simulink model "PotenSchmittwSTM"  (R2024b)
settings: Solver=FixedStepAuto  StartTime=0.0  StopTime=inf  RelTol=1e-3  EnableMultiTasking=on
libraries: fl_lib x16, nesl_utility x10, stm32f4xxblockslib x1
settings Model: STM32="{\"AnalogInput\":[{\"ID\":\"Poten1:1\"},{\"ID\":\"PotenSchmittwSTM:1\"}]}"  Creator=pongn  LastModifiedBy=pongn
settings OptimizationCC: DefaultParameterBehavior=Inlined  EnhancedBackFolding=on  PassReuseOutputArgsAs=Individual arguments  ZeroExternalMemoryAtStartup=off  ZeroInternalMemoryAtStartup=off  MaxStackSize=512  OptimizeBlockOrder=speed  DifferentSizesBufferReuse=on  OptimizationCustomize=off  EfficientTunableParamExpr=on
settings DebuggingCC: ParameterTunabilityLossMsg=error
settings HardwareCC: ProdBitPerPointer=32  ProdBitPerSizeT=32  ProdBitPerPtrDiffT=32  ProdLargestAtomicInteger=Long  ProdLargestAtomicFloat=Double  ProdWordSize=32  ProdLongLongMode=on  ProdHWDeviceType=ARM Compatible->ARM Cortex-M
settings SFSimCC: MATLABDynamicMemAlloc=off
settings RTWCC: Description=Embedded Coder  SystemTargetFile=ert.tlc  HardwareBoard=STM32G4xx Based  TemplateMakefile=ert_default_tmf  Toolchain=GNU Tools for ARM Embedded Processors
settings CodeAppCC: ForceParamTrailComments=on  IgnoreCustomStorageClasses=off  OperatorAnnotations=on  SimulinkDataObjDesc=on  SFDataObjDesc=on  InsertBlockDesc=on
settings ERTTargetCC: TargetLangStandard=C99 (ISO)  CodeReplacementLibrary=ARM Cortex-M  ExtModeTransport=3  ExtModeStaticAlloc=on  ExtModeStaticAllocSize=2048  ExtModeMexFile=ext_xcp  ExtModeIntrfLevel=Level2 - Open

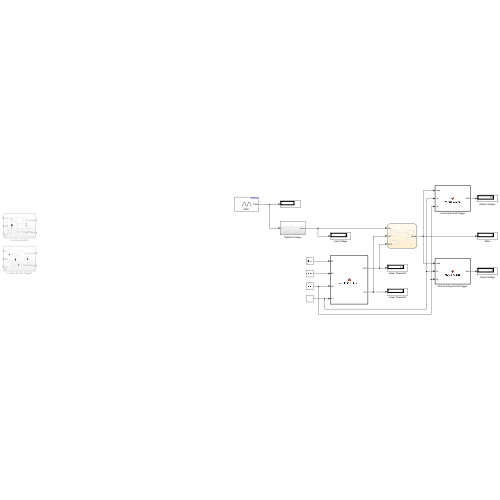
[thumbnail: Simulink's stored preview of the top-level diagram]
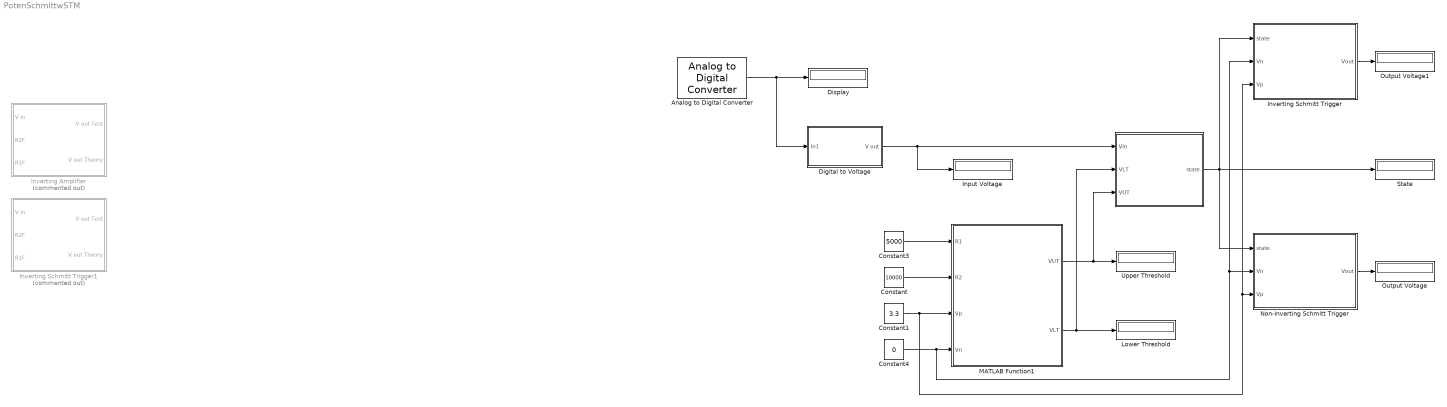
== system PotenSchmittwSTM ==
  " " : Stateflow chart  TreatAsAtomicUnit=on
  Analog to Digital Converter : stm32f4xxblockslib/Analog to Digital Converter  ADCModule=ADC1  ConversionGroup=Regular  TriggerMode=Trigger and read  NumberOfConversions=1  EnableBufferConv=off  BufferLength=1  OutputStatus=off  SampleTime=-1  EnableSimPort=off  hoistedMaskSrc=ECSoC/ECSimCodegen/Analog to Digital Converter
  Constant : Constant  Value=10000
  Constant1 : Constant  Value=3.3
  Constant3 : Constant  Value=5000
  Constant4 : Constant  Value=0
  Digital to Voltage : Subsystem
  Display : Display
  Input Voltage : Display
  Inverting Amplifier : Subsystem  Commented=on
  Inverting Schmitt Trigger : MATLAB Function  TreatAsAtomicUnit=on
  Inverting Schmitt Trigger1 : Subsystem  Commented=on
  Lower Threshold : Display
  MATLAB Function1 : MATLAB Function  TreatAsAtomicUnit=on
  Non-Inverting Schmitt Trigger : MATLAB Function  TreatAsAtomicUnit=on
  Output Voltage : Display
  Output Voltage1 : Display
  State : Display
  Upper Threshold : Display
  wires:
  Analog to Digital Converter/1 -> Digital to Voltage/1(In1), Display/1
  " "/1(state) -> Inverting Schmitt Trigger/1(state), State/1, Non-Inverting Schmitt Trigger/1(state)
  Constant3/1 -> MATLAB Function1/1(R1)
  Constant/1 -> MATLAB Function1/2(R2)
  Constant4/1 -> MATLAB Function1/4(Vn), Inverting Schmitt Trigger/2(Vn), Non-Inverting Schmitt Trigger/2(Vn)
  MATLAB Function1/1(VUT) -> " "/3(VUT), Upper Threshold/1
  MATLAB Function1/2(VLT) -> " "/2(VLT), Lower Threshold/1
  Constant1/1 -> Inverting Schmitt Trigger/3(Vp), Non-Inverting Schmitt Trigger/3(Vp), MATLAB Function1/3(Vp)
  Non-Inverting Schmitt Trigger/1(Vout) -> Output Voltage/1
  Inverting Schmitt Trigger/1(Vout) -> Output Voltage1/1
  Digital to Voltage/1(V out) -> Input Voltage/1, " "/1(Vin)

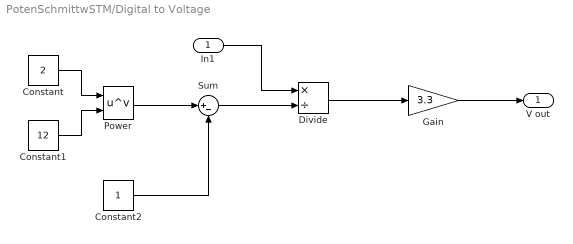
== system PotenSchmittwSTM/Digital to Voltage ==
  In1 : Inport
  Constant : Constant  Value=2
  Constant1 : Constant  Value=12
  Constant2 : Constant
  Divide : Product  Inputs=*/
  Gain : Gain  Gain=3.3
  Power : Math  Operator=pow
  Sum : Sum  Inputs=|+-
  V out : Outport
  wires:
  Constant/1 -> Power/1
  Constant2/1 -> Sum/2
  Sum/1 -> Divide/2
  Power/1 -> Sum/1
  Divide/1 -> Gain/1
  Constant1/1 -> Power/2
  Gain/1 -> V out/1
  In1/1 -> Divide/1

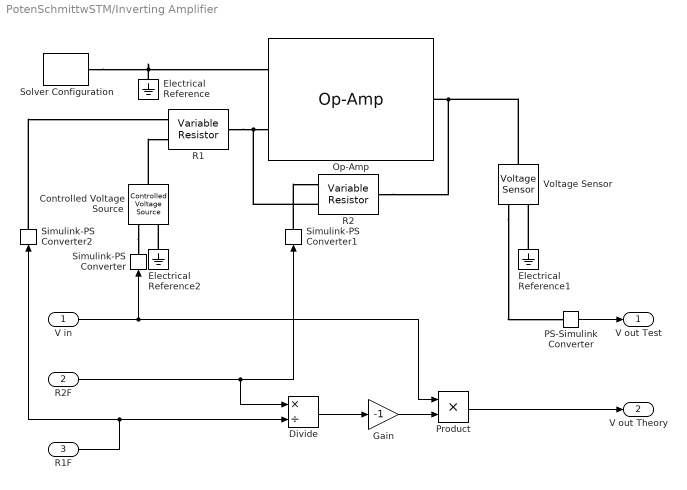
== system PotenSchmittwSTM/Inverting Amplifier ==
  V in : Inport
  R2F : Inport  Port=2
  R1F : Inport  Port=3
  Controlled Voltage Source : fl_lib/Electrical/Electrical Sources/Controlled Voltage Source
  Divide : Product  Inputs=*/
  Electrical Reference : fl_lib/Electrical/Electrical Elements/Electrical Reference
  Electrical Reference1 : fl_lib/Electrical/Electrical Elements/Electrical Reference
  Electrical Reference2 : fl_lib/Electrical/Electrical Elements/Electrical Reference
  Gain : Gain  Gain=-1
  Op-Amp : fl_lib/Electrical/Electrical Elements/Op-Amp  outI_specify=off  outI_priority=None  outI=0 A  outI_nominal_specify=off  outI_nominal_value=1  outI_nominal_unit=A
  PS-Simulink Converter : nesl_utility/PS-Simulink Converter  PhysicalDomain=network_engine_domain  SubClassName=ps_output  LeftPortType=input  RightPortType=output  PseudoPeriodic=off  Frequencies=[]  VectorFormat=inherit  Unit=inherit  AffineConversion=off
  Product : Product
  R1 : fl_lib/Electrical/Electrical Elements/Variable Resistor  Rmin=0 Ohm  thermalEnable=false  thermal_mass=1 J/K  i_specify=off  i_priority=None  i=0 A  i_nominal_specify=off  i_nominal_value=1  i_nominal_unit=A  v_specify=off  v_priority=None  v=0 V  v_nominal_specify=off  v_nominal_value=1  v_nominal_unit=V  T_specify=off  T_priority=None  T=300 K  T_nominal_specify=off  T_nominal_value=1  T_nominal_unit=K
  R2 : fl_lib/Electrical/Electrical Elements/Variable Resistor  Rmin=0 Ohm  thermalEnable=false  thermal_mass=1 J/K  i_specify=off  i_priority=None  i=0 A  i_nominal_specify=off  i_nominal_value=1  i_nominal_unit=A  v_specify=off  v_priority=None  v=0 V  v_nominal_specify=off  v_nominal_value=1  v_nominal_unit=V  T_specify=off  T_priority=None  T=300 K  T_nominal_specify=off  T_nominal_value=1  T_nominal_unit=K
  Simulink-PS Converter : nesl_utility/Simulink-PS Converter  PhysicalDomain=network_engine_domain  SubClassName=ps_input  LeftPortType=input  RightPortType=output  PseudoPeriodic=off  Frequencies=[]  NoiseDistribution=none  NoiseParameters=[]  Unit=1  AffineConversion=off  FilteringAndDerivatives=provide  SimscapeFilterOrder=1  InputFilterTimeConstant=0.001  UdotUserProvided=0
  Simulink-PS Converter1 : nesl_utility/Simulink-PS Converter  PhysicalDomain=network_engine_domain  SubClassName=ps_input  LeftPortType=input  RightPortType=output  PseudoPeriodic=off  Frequencies=[]  NoiseDistribution=none  NoiseParameters=[]  Unit=1  AffineConversion=off  FilteringAndDerivatives=provide  SimscapeFilterOrder=1  InputFilterTimeConstant=0.001  UdotUserProvided=0
  Simulink-PS Converter2 : nesl_utility/Simulink-PS Converter  PhysicalDomain=network_engine_domain  SubClassName=ps_input  LeftPortType=input  RightPortType=output  PseudoPeriodic=off  Frequencies=[]  NoiseDistribution=none  NoiseParameters=[]  Unit=1  AffineConversion=off  FilteringAndDerivatives=provide  SimscapeFilterOrder=1  InputFilterTimeConstant=0.001  UdotUserProvided=0
  Solver Configuration : nesl_utility/Solver Configuration  PhysicalDomain=network_engine_domain  SubClassName=solver  LeftPortType=input  RightPortType=generic  Tones=[]  Harmonics=[]  SimulateNoise=off  Profile=off  UseLocalSampling=off  EnableSwitchedLinearOptims=on  FrequencyDomain=off  UseCCode=off  RelTol=0.001  AbsTol=0.001  MinStep=1e-09  ToWorkspace=off  RevertToSquareIcSolve=off  NumHomotopyIterations=100  PhasorMode=off  PhasorModeNumHarmonics=1  ConsistencySolver=NEWTON_XTOL_AFTER_FTOL  IndexReductionMethod=DerivativeReplacement  DoDC=off  ResidualTolerance=1e-09  ConsistencyTolSource=GLOBAL  ConsistencyAbsTol=0.001  ConsistencyRelTol=0.001  ConsistencyTolFactor=0.001  UseLocalSolver=off  LocalSolverChoice=NE_BACKWARD_EULER_ADVANCER  ResolveIndetEquations=on  FunctionEvalNumThread=1  LocalSolverSampleTime=0.001  DoFixedCost=off  MaxNonlinIter=3  MaxModeIter=2  ComputeImpulses=off  ImpulseIterations=2  LinearAlgebra=auto  LinearAlgebraNumThread=0  EquationFormulation=NE_TIME_EF  DelaysMemoryBudget=1024  AutomaticFiltering=on  FilteringTimeConstant=0.001  PartitionStorageMethod=AS_NEEDED  PartitionMemoryBudget=1024  PartitionMethod=ROBUST  MultibodyUseLocalSolver=off  MultibodyLocalSolverChoice=ODE1  MultibodyLocalSolverSampleTime=0.001
  Voltage Sensor : fl_lib/Electrical/Electrical Sensors/Voltage Sensor
  V out Test : Outport
  V out Theory : Outport  Port=2
  wires:
  Divide/1 -> Gain/1
  Gain/1 -> Product/2
  V in/1 -> Simulink-PS Converter/1, Product/1
  Product/1 -> V out Theory/1
  R2F/1 -> Simulink-PS Converter1/1, Divide/1
  R1F/1 -> Divide/2, Simulink-PS Converter2/1
  PS-Simulink Converter/1 -> V out Test/1
  connections:
  Voltage Sensor/LConn1 -- Op-Amp/RConn1 -- R2/RConn1
  R1/RConn1 -- Op-Amp/LConn2 -- R2/LConn2
  Solver Configuration/RConn1 -- Electrical Reference/LConn1 -- Op-Amp/LConn1
  Voltage Sensor/RConn1 -- PS-Simulink Converter/LConn1
  Electrical Reference1/LConn1 -- Voltage Sensor/RConn2
  Controlled Voltage Source/RConn1 -- Simulink-PS Converter/RConn1
  Controlled Voltage Source/LConn1 -- R1/LConn2
  Electrical Reference2/LConn1 -- Controlled Voltage Source/RConn2
  Simulink-PS Converter1/RConn1 -- R2/LConn1
  Simulink-PS Converter2/RConn1 -- R1/LConn1

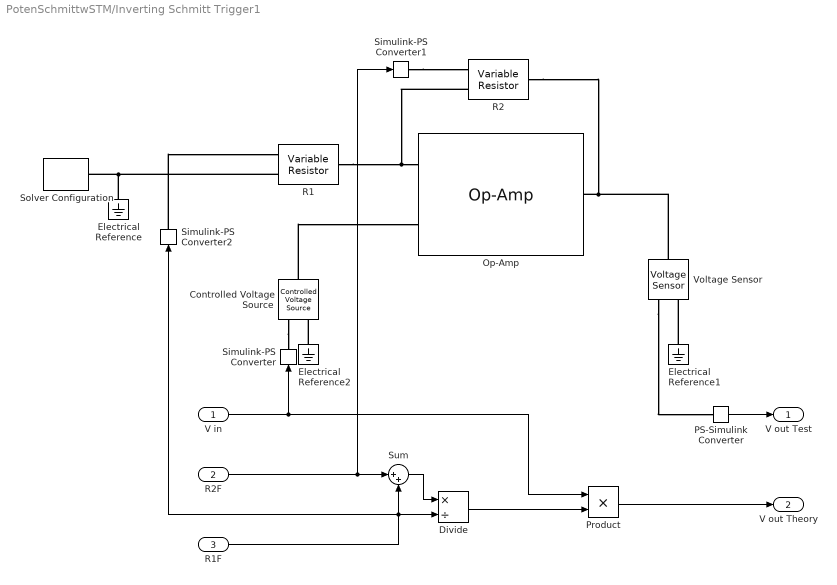
== system PotenSchmittwSTM/Inverting Schmitt Trigger1 ==
  V in : Inport
  R2F : Inport  Port=2
  R1F : Inport  Port=3
  Controlled Voltage Source : fl_lib/Electrical/Electrical Sources/Controlled Voltage Source
  Divide : Product  Inputs=*/
  Electrical Reference : fl_lib/Electrical/Electrical Elements/Electrical Reference
  Electrical Reference1 : fl_lib/Electrical/Electrical Elements/Electrical Reference
  Electrical Reference2 : fl_lib/Electrical/Electrical Elements/Electrical Reference
  Op-Amp : fl_lib/Electrical/Electrical Elements/Op-Amp  outI_specify=off  outI_priority=None  outI=0 A  outI_nominal_specify=off  outI_nominal_value=1  outI_nominal_unit=A
  PS-Simulink Converter : nesl_utility/PS-Simulink Converter  PhysicalDomain=network_engine_domain  SubClassName=ps_output  LeftPortType=input  RightPortType=output  PseudoPeriodic=off  Frequencies=[]  VectorFormat=inherit  Unit=inherit  AffineConversion=off
  Product : Product
  R1 : fl_lib/Electrical/Electrical Elements/Variable Resistor  Rmin=0 Ohm  thermalEnable=false  thermal_mass=1 J/K  i_specify=off  i_priority=None  i=0 A  i_nominal_specify=off  i_nominal_value=1  i_nominal_unit=A  v_specify=off  v_priority=None  v=0 V  v_nominal_specify=off  v_nominal_value=1  v_nominal_unit=V  T_specify=off  T_priority=None  T=300 K  T_nominal_specify=off  T_nominal_value=1  T_nominal_unit=K
  R2 : fl_lib/Electrical/Electrical Elements/Variable Resistor  Rmin=0 Ohm  thermalEnable=false  thermal_mass=1 J/K  i_specify=off  i_priority=None  i=0 A  i_nominal_specify=off  i_nominal_value=1  i_nominal_unit=A  v_specify=off  v_priority=None  v=0 V  v_nominal_specify=off  v_nominal_value=1  v_nominal_unit=V  T_specify=off  T_priority=None  T=300 K  T_nominal_specify=off  T_nominal_value=1  T_nominal_unit=K
  Simulink-PS Converter : nesl_utility/Simulink-PS Converter  PhysicalDomain=network_engine_domain  SubClassName=ps_input  LeftPortType=input  RightPortType=output  PseudoPeriodic=off  Frequencies=[]  NoiseDistribution=none  NoiseParameters=[]  Unit=1  AffineConversion=off  FilteringAndDerivatives=provide  SimscapeFilterOrder=1  InputFilterTimeConstant=0.001  UdotUserProvided=0
  Simulink-PS Converter1 : nesl_utility/Simulink-PS Converter  PhysicalDomain=network_engine_domain  SubClassName=ps_input  LeftPortType=input  RightPortType=output  PseudoPeriodic=off  Frequencies=[]  NoiseDistribution=none  NoiseParameters=[]  Unit=1  AffineConversion=off  FilteringAndDerivatives=provide  SimscapeFilterOrder=1  InputFilterTimeConstant=0.001  UdotUserProvided=0
  Simulink-PS Converter2 : nesl_utility/Simulink-PS Converter  PhysicalDomain=network_engine_domain  SubClassName=ps_input  LeftPortType=input  RightPortType=output  PseudoPeriodic=off  Frequencies=[]  NoiseDistribution=none  NoiseParameters=[]  Unit=1  AffineConversion=off  FilteringAndDerivatives=provide  SimscapeFilterOrder=1  InputFilterTimeConstant=0.001  UdotUserProvided=0
  Solver Configuration : nesl_utility/Solver Configuration  PhysicalDomain=network_engine_domain  SubClassName=solver  LeftPortType=input  RightPortType=generic  Tones=[]  Harmonics=[]  SimulateNoise=off  Profile=off  UseLocalSampling=off  EnableSwitchedLinearOptims=on  FrequencyDomain=off  UseCCode=off  RelTol=0.001  AbsTol=0.001  MinStep=1e-09  ToWorkspace=off  RevertToSquareIcSolve=off  NumHomotopyIterations=100  PhasorMode=off  PhasorModeNumHarmonics=1  ConsistencySolver=NEWTON_XTOL_AFTER_FTOL  IndexReductionMethod=DerivativeReplacement  DoDC=off  ResidualTolerance=1e-09  ConsistencyTolSource=GLOBAL  ConsistencyAbsTol=0.001  ConsistencyRelTol=0.001  ConsistencyTolFactor=0.001  UseLocalSolver=off  LocalSolverChoice=NE_BACKWARD_EULER_ADVANCER  ResolveIndetEquations=on  FunctionEvalNumThread=1  LocalSolverSampleTime=0.001  DoFixedCost=off  MaxNonlinIter=3  MaxModeIter=2  ComputeImpulses=off  ImpulseIterations=2  LinearAlgebra=auto  LinearAlgebraNumThread=0  EquationFormulation=NE_TIME_EF  DelaysMemoryBudget=1024  AutomaticFiltering=on  FilteringTimeConstant=0.001  PartitionStorageMethod=AS_NEEDED  PartitionMemoryBudget=1024  PartitionMethod=ROBUST  MultibodyUseLocalSolver=off  MultibodyLocalSolverChoice=ODE1  MultibodyLocalSolverSampleTime=0.001
  Sum : Sum  Inputs=|++
  Voltage Sensor : fl_lib/Electrical/Electrical Sensors/Voltage Sensor
  V out Test : Outport
  V out Theory : Outport  Port=2
  wires:
  R2F/1 -> Simulink-PS Converter1/1, Sum/1
  Sum/1 -> Divide/1
  R1F/1 -> Divide/2, Simulink-PS Converter2/1, Sum/2
  PS-Simulink Converter/1 -> V out Test/1
  Product/1 -> V out Theory/1
  V in/1 -> Product/1, Simulink-PS Converter/1
  Divide/1 -> Product/2
  connections:
  Controlled Voltage Source/LConn1 -- Op-Amp/LConn2
  R2/LConn2 -- R1/RConn1 -- Op-Amp/LConn1
  Simulink-PS Converter2/RConn1 -- R1/LConn1
  Simulink-PS Converter1/RConn1 -- R2/LConn1
  Electrical Reference2/LConn1 -- Controlled Voltage Source/RConn2
  Controlled Voltage Source/RConn1 -- Simulink-PS Converter/RConn1
  Electrical Reference1/LConn1 -- Voltage Sensor/RConn2
  Voltage Sensor/RConn1 -- PS-Simulink Converter/LConn1
  R1/LConn2 -- Solver Configuration/RConn1 -- Electrical Reference/LConn1
  R2/RConn1 -- Op-Amp/RConn1 -- Voltage Sensor/LConn1

== matlab function PotenSchmittwSTM/MATLAB Function1 ==
  data: R1 input; R2 input; Vp input; VUT output; Vn input; VLT output
% VUT : Upper Threshold Voltage
% VLT : Lower Threshold Voltage
% Vout : Output Voltage
% Vin : Input Voltage
% R1 : 1st Resistor
% R2 : 2nd Resistor
% Vp : Op-Amp V+
% Vn : Op-Amp V-

function [VUT, VLT] = VariableCalculation(R1,R2,Vp, Vn)

VUT = Vp * (R2 / (R1 + R2));
VLT = Vn * (R2 / (R1 + R2));

== matlab function PotenSchmittwSTM/Non-Inverting Schmitt Trigger ==
  data: state input; Vn input; Vp input; Vout output
% VUT : Upper Threshold Voltage
% VLT : Lower Threshold Voltage
% Vout : Output Voltage
% Vin : Input Voltage
% R1 : 1st Resistor
% R2 : 2nd Resistor
% Vp : Op-Amp V+
% Vn : Op-Amp V-

function Vout = VoutCalculation(state, Vn, Vp)
Vout = 0;

if state == 1
    Vout = Vp;
elseif state == 0
    Vout = Vn;
end

== stateflow chart PotenSchmittwSTM/  ==
  state Initial
    state = 0;
  state LessThanVLT
    during:
    state = 0;
  state MoreThanVUT
    during:
    state = 1;
  (default) -> Initial
  Initial -> LessThanVLT [order 1] : [state == 0]
  MoreThanVUT -> LessThanVLT : [Vin <= VLT]
  LessThanVLT -> MoreThanVUT : [Vin >= VUT]
  Initial -> MoreThanVUT [order 2] : [state == 1]
  data: Vin input; VLT input; VUT input; state output

== matlab function PotenSchmittwSTM/Inverting Schmitt Trigger ==
  data: state input; Vn input; Vp input; Vout output
% VUT : Upper Threshold Voltage
% VLT : Lower Threshold Voltage
% Vout : Output Voltage
% Vin : Input Voltage
% R1 : 1st Resistor
% R2 : 2nd Resistor
% Vp : Op-Amp V+
% Vn : Op-Amp V-

function Vout = VoutCalculation(state, Vn, Vp)
Vout = 0;

if state == 1
    Vout = Vn;
elseif state == 0
    Vout = Vp;
end
